simulink model "observer"  (R2023a)
settings: Solver=VariableStepAuto  StartTime=0.0  StopTime=30  RelTol=1e-3
model workspace (MAT data in the model file):
  initial_position = 1
  initial_velocity = 1
settings Model: Creator=asus  LastModifiedBy=asus

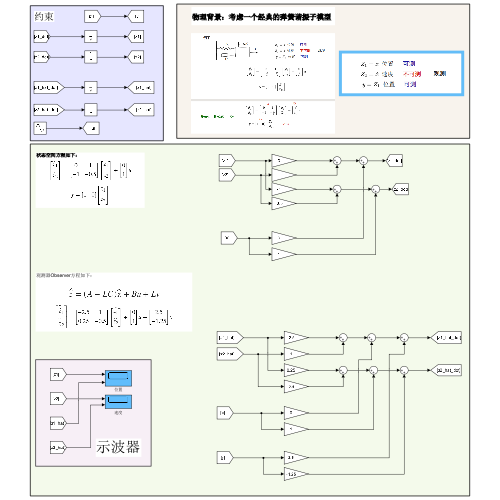
[thumbnail: Simulink's stored preview of the top-level diagram]
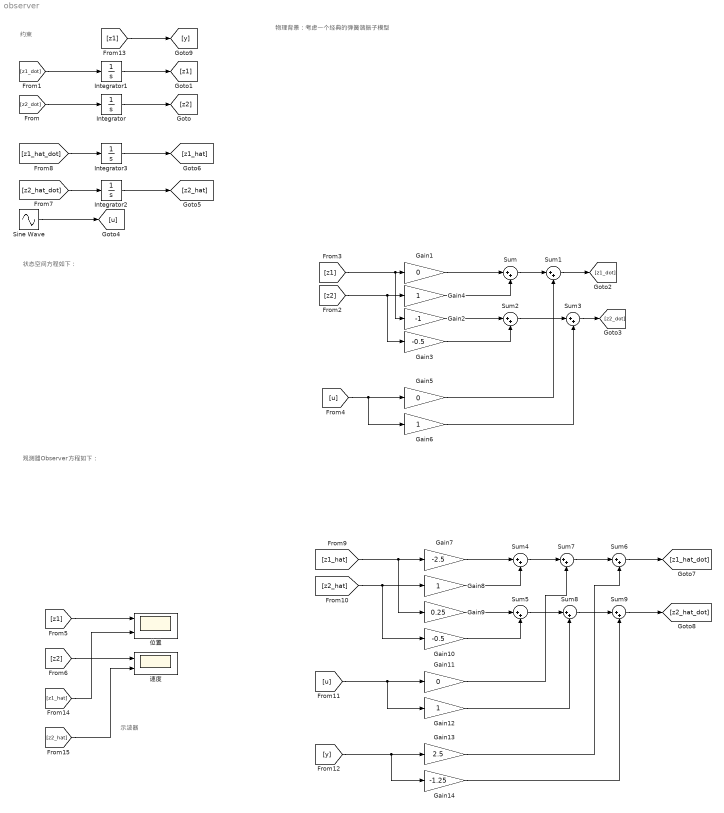
== system observer ==
  note: 示波器
  note: 观测器Observer方程如下：
  note: 状态空间方程如下：
  note: 约束
  note: 物理背景：考虑一个经典的弹簧谐振子模型
  Gain1 : Gain  Gain=0
  Gain10 : Gain  Gain=-0.5
  Gain11 : Gain  Gain=0
  Gain{4,6,8,12} (4 alike) : Gain
  Gain13 : Gain  Gain=2.5
  Gain14 : Gain  Gain=-1.25
  Gain2 : Gain  Gain=-1
  Gain3 : Gain  Gain=-0.5
  Gain5 : Gain  Gain=0
  Gain7 : Gain  Gain=-2.5
  Gain9 : Gain  Gain=0.25
  Integrator : Integrator  InitialCondition=initial_velocity
  Integrator1 : Integrator  InitialCondition=initial_position
  Integrator2 : Integrator
  Integrator3 : Integrator
  Sine Wave : Sin  Amplitude=2  Frequency=2*pi*10  SampleTime=0
  Sum{,1..9} (10 alike) : Sum  Inputs=|++
  位置 : Scope  NumInputPorts=2
  速度 : Scope  NumInputPorts=2
  wires:
  [z2_dot] -> Integrator/1
  Integrator/1 -> [z2]
  [z1_dot] -> Integrator1/1
  Integrator1/1 -> [z1]
  [z1] -> Gain2/1, Gain1/1
  [z2] -> Gain3/1, Gain4/1
  Gain1/1 -> Sum/1
  Gain4/1 -> Sum/2
  Sum1/1 -> [z1_dot]
  Sum/1 -> Sum1/1
  Gain2/1 -> Sum2/1
  Gain3/1 -> Sum2/2
  [u] -> Gain6/1, Gain5/1
  Gain5/1 -> Sum1/2
  Sum3/1 -> [z2_dot]
  Gain6/1 -> Sum3/2
  Sum2/1 -> Sum3/1
  [z1] -> 位置/1
  [z2] -> 速度/1
  [z1_hat_dot] -> Integrator3/1
  Integrator3/1 -> [z1_hat]
  [z2_hat_dot] -> Integrator2/1
  Integrator2/1 -> [z2_hat]
  [z1_hat] -> Gain9/1, Gain7/1
  [z2_hat] -> Gain10/1, Gain8/1
  [u] -> Gain11/1, Gain12/1
  [y] -> Gain14/1, Gain13/1
  Gain7/1 -> Sum4/1
  Gain8/1 -> Sum4/2
  Gain9/1 -> Sum5/1
  Gain10/1 -> Sum5/2
  Sum6/1 -> [z1_hat_dot]
  Sum4/1 -> Sum7/1
  Gain11/1 -> Sum7/2
  Sum5/1 -> Sum8/1
  Gain12/1 -> Sum8/2
  Sum7/1 -> Sum6/1
  Gain13/1 -> Sum6/2
  Gain14/1 -> Sum9/2
  Sum9/1 -> [z2_hat_dot]
  [z1] -> [y]
  [z1_hat] -> 位置/2
  [z2_hat] -> 速度/2
  Sine Wave/1 -> [u]
  Sum8/1 -> Sum9/1
